simulink model "HITL"  (R2020a)
settings: Solver=ode4  StartTime=0.0  StopTime=100  FixedStep=0.02  RelTol=1e-3  EnableMultiTasking=on
values from neighbouring files (symbols this model uses):
  g = data(5); Quad.b = data(6); Quad.d = data(7); Quad.l = data(8)    [Quad1.m]
undefined symbols (not defined in the file or in its folder): sigbuilder_block
libraries: aerolibutil x10, simulink x9, sharedutil x3, dspindex x2, dspmathops x2, vrlib x1
(part 2 of 2)

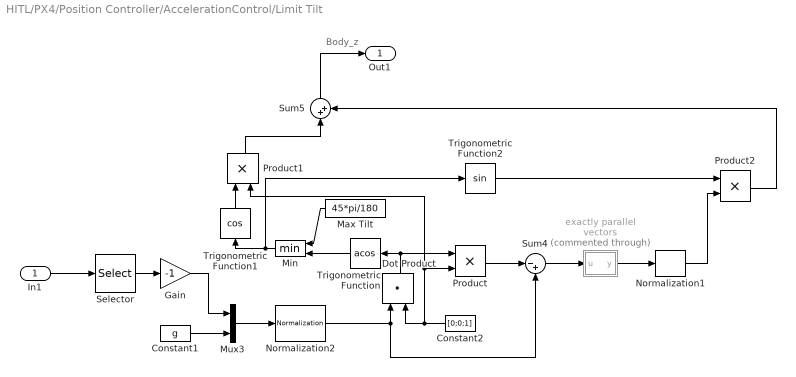
== system HITL/PX4/Position Controller/AccelerationControl/Limit Tilt ==
  note: Body_z
  In1 : Inport
  Constant1 : Constant  Value=g
  Constant2 : Constant  Value=[0;0;1]
  Dot Product : DotProduct  InputSameDT=on  OutDataTypeStr=Inherit: Inherit via internal rule
  Gain : Gain  Gain=-1
  Max Tilt : Constant  Value=45*pi/180
  Min : MinMax  Inputs=2
  Mux3 : Mux  Inputs=2
  Normalization1 : dspmathops/Normalization  NormType=2-norm  Bias=1e-10  NormOver=Each column  Dimension=1  roundingMode=Floor  overflowMode=off  accumDataTypeStr=Inherit: Same as product output  accumLastDataTypeStr=Inherit: Same as product output  outputDataTypeStr=Inherit: Same as product output  outputMin=[]  outputMax=[]  outputLastDataTypeStr=Inherit: Same as product output
  Normalization2 : dspmathops/Normalization  NormType=2-norm  Bias=1e-10  NormOver=Each column  Dimension=1  roundingMode=Floor  overflowMode=off  accumDataTypeStr=Inherit: Same as product output  accumLastDataTypeStr=Inherit: Same as product output  outputDataTypeStr=Inherit: Same as product output  outputMin=[]  outputMax=[]  outputLastDataTypeStr=Inherit: Same as product output
  Product : Product
  Product1 : Product
  Product2 : Product
  Selector : Selector  InputPortWidth=3  IndexOptions=Index vector (dialog)  Indices=[1 2]  OutputSizes=1
  Sum4 : Sum  Inputs=|-+
  Sum5 : Sum  Inputs=|++
  Trigonometric Function : Trigonometry  Operator=acos
  Trigonometric Function1 : Trigonometry  Operator=cos
  Trigonometric Function2 : Trigonometry
  exactly parallel vectors : MATLAB Function  Commented=through  TreatAsAtomicUnit=on
  Out1 : Outport
  wires:
  Trigonometric Function2/1 -> Product2/1
  Product1/1 -> Sum5/1
  Mux3/1 -> Normalization2/1
  Min/1 -> Trigonometric Function1/1, Trigonometric Function2/1
  Trigonometric Function1/1 -> Product1/1
  Trigonometric Function/1 -> Min/2
  Constant2/1 -> Dot Product/2, Product/2, Product1/2
  Normalization2/1 -> Sum4/2, Dot Product/1
  Dot Product/1 -> Product/1, Trigonometric Function/1
  Product2/1 -> Sum5/2
  Constant1/1 -> Mux3/2
  Selector/1 -> Gain/1
  Product/1 -> Sum4/1
  In1/1 -> Selector/1
  Sum5/1 -> Out1/1
  Gain/1 -> Mux3/1
  Sum4/1 -> exactly parallel vectors/1(u)
  exactly parallel vectors/1(y) -> Normalization1/1
  Max Tilt/1 -> Min/1
  Normalization1/1 -> Product2/2

== system HITL/PX4/Position Controller/ThrustToAttitude/Thrust To Attitude ==
  thr_sp : Inport
  yaw_sp : Inport  Port=2
  3x3 Cross Product : sharedutil/3x3 Cross Product  aMode=aMode
      settings: SourceProductBaseCode=AE,PW,MT,VE,VP
  3x3 Cross Product1 : sharedutil/3x3 Cross Product  aMode=aMode
      settings: SourceProductBaseCode=AE,PW,MT,VE,VP
  Gain : Gain  Gain=-1
  Keep Nose to front & normalize : MATLAB Function  TreatAsAtomicUnit=on
  Normalize : MATLAB Function  TreatAsAtomicUnit=on
  y_c : Subsystem
  Rx : Outport  PortDimensions=3
  Ry : Outport  Port=2  PortDimensions=3
  Rz : Outport  Port=3  PortDimensions=3
  wires:
  y_c/1(y_c) -> 3x3 Cross Product/1
  3x3 Cross Product1/1 -> Ry/1  "y_body_desired"
  Normalize/1(y) -> Keep Nose to front & normalize/2(Z_body), 3x3 Cross Product1/1, Rz/1, 3x3 Cross Product/2  "Z_body_desired"
  yaw_sp/1 -> y_c/1(psi_req)
  Keep Nose to front & normalize/1(y) -> Rx/1, 3x3 Cross Product1/2
  thr_sp/1 -> Gain/1
  3x3 Cross Product/1 -> Keep Nose to front & normalize/1(u)  "X_body_desired"
  Gain/1 -> Normalize/1(u)

== system HITL/PX4/Position Controller/ThrustToAttitude/Thrust To Attitude/y_c ==
  psi_req : Inport
  Constant : Constant  Value=0
  Display : Display
  Display1 : Display
  Gain : Gain  Gain=-1
  Mux : Mux  Inputs=3
  Trigonometric Function : Trigonometry
  Trigonometric Function1 : Trigonometry  Operator=cos
  y_c : Outport
  wires:
  Trigonometric Function1/1 -> Display1/1, Mux/2
  Constant/1 -> Mux/3
  Mux/1 -> y_c/1
  Trigonometric Function/1 -> Display/1, Gain/1
  Gain/1 -> Mux/1
  psi_req/1 -> Trigonometric Function1/1, Trigonometric Function/1

== matlab function HITL/PX4/Position Controller/ThrustToAttitude/Thrust To Attitude/Normalize ==
  data: u input; y output
function y = fcn(u)
if norm(u)^2 < 1.1920929e-7
    u(3) = 1;
end
y = u / norm(u);
end

== matlab function HITL/PX4/Position Controller/AccelerationControl/Limit Tilt/exactly parallel vectors ==
  data: u input; y output
function y = fcn(u)
if norm(u)^2 < 1.1920929e-7
    u(1)=1;
end
y=u;

== matlab function HITL/PX4/Attitude_Controller2/Check for corner case ==
  data: qd_red input; qd_cmd output; qd input; q input
function qd_cmd = fcn(qd_red,qd,q)
if abs(qd_red(2))> (1-1e-5) || abs(qd_red(3))> (1-1e-5)
    qd_cmd = qd;
else
    qd_cmd = quatmultiply(q',qd_red')';
end
end

== matlab function HITL/PX4/Attitude_Controller2/MATLAB Function ==
  data: q input; q_can output
function q_can = fcn(q)
q_can = q;
for i =1:4
    if abs(q(i)) > 1e-7
        q_can = sign(q_can(i))*q_can;
    end
end
end

== matlab function HITL/PX4/Attitude_Controller2/MATLAB Function1 ==
  data: q input; q_can output
function q_can = fcn(q)
q_can = q;
for i =1:4
    if abs(q(i)) > 1e-7
        q_can = sign(q_can(i))*q_can;
    end
end
end

== matlab function HITL/PX4/Attitude_Controller2/Q to DCM (z_comp) ==
  data: u input; y output
function y = fcn(u)
q0 = u(1); q1 = u(2); q2 = u(3); q3 = u(4);

R13 = 2*(q0*q2 + q1*q3);


R23 = 2*(q2*q3 - q0*q1);

R33 = q0^2 - q1^2 - q2^2 + q3^2;

 y= [R13 R23 R33];

== matlab function HITL/PX4/Attitude_Controller2/Q to DCM (Z_comp) ==
  data: u input; y output
function y = fcn(u)
q0 = u(1); q1 = u(2); q2 = u(3); q3 = u(4);

R13 = 2*(q0*q2 + q1*q3);


R23 = 2*(q2*q3 - q0*q1);

R33 = q0^2 - q1^2 - q2^2 + q3^2;

 y= [R13 R23 R33];

== matlab function HITL/PX4/Attitude_Controller2/Q to DCM (z_comp.) ==
  data: u input; y output
function y = fcn(u)
q0 = u(1); q1 = u(2); q2 = u(3); q3 = u(4);

R13 = 2*(q0*q2 + q1*q3);


R23 = 2*(q2*q3 - q0*q1);

R33 = q0^2 - q1^2 - q2^2 + q3^2;

 y= [R13 R23 R33];

== matlab function HITL/PX4/Attitude_Controller2/Quaternion from 2 vectors ==
  data: Z_cur input; qd_red output; Z_des input
function qd_red = fun(Z_cur,Z_des)
coder.extrinsic('vrrotvec')
qd_red = [1;0;0;0];
% eps = 1e-5;
% cr = cross(Z_cur,Z_des);
% dt = dot(Z_cur,Z_des);
% if norm(cr) < eps && dt < 0
%     cr = abs(Z_cur);
%     if cr(1) < cr(2)
%         if cr(1) < cr(3)
%             cr = [1;0;0];
%         else
%             cr = [0;0;1];
%         end
%     else
%         if cr(2) < cr(3)
%             cr = [0;1;0];
%         else
%             cr = [0;0;1];
%         end
%     end
%     qd_red(1) = 0;
%     cr = cross(Z_cur,cr);
% else
%     qd_red(1) = dt + sqrt((norm(Z_cur))^2*(norm(Z_des))^2);
% end
% qd_red(2) = cr(1);
% qd_red(3) = cr(2);
% qd_red(4) = cr(3);
% qd_red = qd_red / norm(qd_red);
q=quatnormalize(vrrotvec(Z_cur,Z_des));
qd_red =[q(4),q(1),q(2),q(3)];
end

== matlab function HITL/PX4/Attitude Controller/Check for corner case ==
  data: qd_red input; qd_cmd output; qd input; q input
function qd_cmd = fcn(qd_red,qd,q)
if abs(qd_red(2))> (1-1e-5) || abs(qd_red(3))> (1-1e-5)
    qd_cmd = qd;
else
    qd_cmd = quatmultiply(q',qd_red')';
end
end

== matlab function HITL/PX4/Position Controller/ThrustToAttitude/Rotaion Matrix To Q ==
  data: u input; y output
function y = fcn(u)
R11=u(1,1);R12=u(1,2);R13=u(1,3);
R21=u(2,1);R22=u(2,2);R23=u(2,3);
R31=u(3,1);R32=u(3,2);R33=u(3,3);
q0 = sqrt(1+ R11 + R22 + R33)/2;
q1 = (R32 - R23)/4/q0;
q2 = (R13 - R31)/4/q0;
q3 = (R21 - R12)/4/q0;

y = [q0;q1;q2;q3];

== matlab function HITL/PX4/Mixer/Float Epsilon  ==
  data: u input; y output
function y = fcn(u)
if abs(u(1))< 1.1920929e-7
    u(1)=0;
end
if abs(u(2))< 1.1920929e-7
    u(2)=0;
end
if abs(u(3))< 1.1920929e-7
    u(3)=0;
end
if abs(u(4))< 1.1920929e-7
    u(4)=0;
end
y=u;

== matlab function HITL/PX4/Position Controller/AccelerationControl/XY - Saturation ==
  data: u1 input; y1 output; u2 input; y2 output; u_max_squared input
function [y1,y2] = fcn(u1,u2,u_max_squared)
u_max = 0;
if u_max_squared > 0
    u_max= sqrt(u_max_squared);
end
Norm = norm([u1 u2]);
if Norm > u_max
    y1 = u1/Norm*u_max;
    y2 = u2/Norm*u_max;
else
    y1 = u1;
    y2 = u2;
end
end

== matlab function HITL/PX4/Attitude Controller/Q to Rottion Matrix ==
  data: u input; y output
function y = fcn(u)
q0 = u(1); q1 = u(2); q2 = u(3); q3 = u(4);
R11 = q0^2 + q1^2 - q2^2 - q3^2;
R12 = 2*(q1*q2 - q0*q3);
R13 = 2*(q0*q2 + q1*q3);

R21 = 2*(q1*q2 + q0*q3);
R22 = q0^2 - q1^2 + q2^2 - q3^2;
R23 = 2*(q2*q3 - q0*q1);

R31 = 2*(q1*q3 - q0*q2);
R32 = 2*(q0*q1 + q2*q3);
R33 = q0^2 - q1^2 - q2^2 + q3^2;

y= [R11 R12 R13;
    R21 R22 R23;
    R31 R32 R33;];

== matlab function HITL/PX4/Attitude Controller/Q to Rottion Matrix1 ==
  data: u input; y output
function y = fcn(u)
q0 = u(1); q1 = u(2); q2 = u(3); q3 = u(4);
R11 = q0^2 + q1^2 - q2^2 - q3^2;
R12 = 2*(q1*q2 - q0*q3);
R13 = 2*(q0*q2 + q1*q3);

R21 = 2*(q1*q2 + q0*q3);
R22 = q0^2 - q1^2 + q2^2 - q3^2;
R23 = 2*(q2*q3 - q0*q1);

R31 = 2*(q1*q3 - q0*q2);
R32 = 2*(q0*q1 + q2*q3);
R33 = q0^2 - q1^2 - q2^2 + q3^2;

y= [R11 R12 R13;
    R21 R22 R23;
    R31 R32 R33;];

== matlab function HITL/PX4/Position Controller/ThrustToAttitude/Thrust To Attitude/Keep Nose to front & normalize ==
  data: u input; y output; Z_body input
function y = fcn(u, Z_body)
if Z_body(3)<0
    u = -u;
end
if abs(Z_body(3))<1e-6
    u = [0;0;1];
end
y = u /norm(u);
end

== matlab function HITL/PX4/Attitude Controller/Float epsilon ==
  data: u input; y output
function y = fcn(u)
if abs(u(1))< 1e-7
    u(1)=0;
end
if abs(u(2))< 1e-7
    u(2)=0;
end
if abs(u(3))< 1e-7
    u(3)=0;
end
if abs(u(4))< 1e-7
    u(4)=0;
end
y=u;

== matlab function HITL/PX4/Attitude Controller/Float Epsilon ==
  data: u input; y output
function y = fcn(u)
if abs(u(1))< 1e-7
    u(1)=0;
end
if abs(u(2))< 1e-7
    u(2)=0;
end
if abs(u(3))< 1e-7
    u(3)=0;
end
if abs(u(4))< 1e-7
    u(4)=0;
end
y=u;

== matlab function HITL/PX4/Attitude Controller/Quaternion from 2 vectors ==
  data: Z_cur input; qd_red output; Z_des input
function qd_red = fun(Z_cur,Z_des)
qd_red = [1;0;0;0];
eps = 1e-5;
cr = cross(Z_cur,Z_des);
dt = dot(Z_cur,Z_des);
if norm(cr) < eps && dt < 0
    cr = abs(Z_cur);
    if cr(1) < cr(2)
        if cr(1) < cr(3)
            cr = [1;0;0];
        else
            cr = [0;0;1];
        end
    else
        if cr(2) < cr(3)
            cr = [0;1;0];
        else
            cr = [0;0;1];
        end
    end
    qd_red(1) = 0;
    cr = cross(Z_cur,cr);
else
    qd_red(1) = dt + sqrt((norm(Z_cur))^2*(norm(Z_des))^2);
end
qd_red(2) = cr(1);
qd_red(3) = cr(2);
qd_red(4) = cr(3);
qd_red = qd_red / norm(qd_red);
end

== matlab function HITL/Euler to Q ==
  data: u input; y output
function y = fcn(u)
y = [cos(u(1)/2)*cos(u(2)/2)*cos(u(3)/2)+sin(u(1)/2)*sin(u(2)/2)*sin(u(3)/2);
    -cos(u(1)/2)*sin(u(2)/2)*sin(u(3)/2)+sin(u(1)/2)*cos(u(2)/2)*cos(u(3)/2);
    cos(u(1)/2)*sin(u(2)/2)*cos(u(3)/2)+sin(u(1)/2)*cos(u(2)/2)*sin(u(3)/2);
    cos(u(1)/2)*cos(u(2)/2)*sin(u(3)/2)-sin(u(1)/2)*sin(u(2)/2)*cos(u(3)/2)];
